simulink model "ComControleRobustoSemIntegral"  (R2024a)
settings: Solver=ode3  StartTime=0.0  StopTime=10  FixedStep=0.001  MaxStep=10^-3  RelTol=1e-6  AbsTol=10^-6
values from neighbouring files (symbols this model uses):
  A = [-807.7,  222.7,    0,      0,       0 ... (first row only)    [test.m]
  B = [-1073,  -1684,  824.5 ... (first row only)    [test.m]
  C = [21.93,  -18.87,  144.4,  -100.7,  13.85 ... (first row only)    [test.m]
undefined symbols (not defined in the file or in its folder): D, K, sigbuilder_block
libraries: simulink_extras x1
settings Model: Creator=Vilson Wenis Belle  LastModifiedBy=wenis
settings SolverCC: AlgebraicLoopSolver=TrustRegion
settings DebuggingCC: UnconnectedInputMsg=warning  UnconnectedOutputMsg=warning  UnconnectedLineMsg=warning
settings ModelReferenceCC: EnableRefExpFcnMdlSchedulingChecks=on
settings RTWCC: GPUComputeCapability=3.5  DLArmComputeVersion=19.05

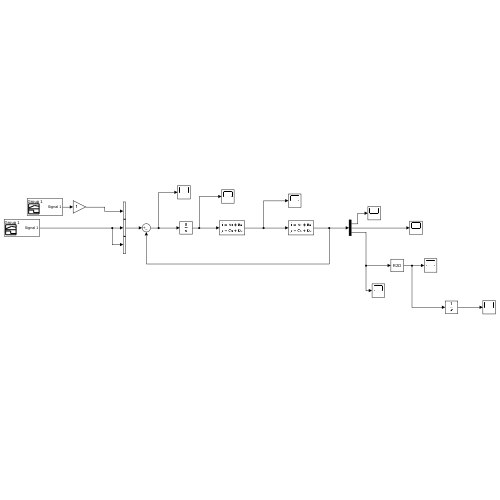
[thumbnail: Simulink's stored preview of the top-level diagram]
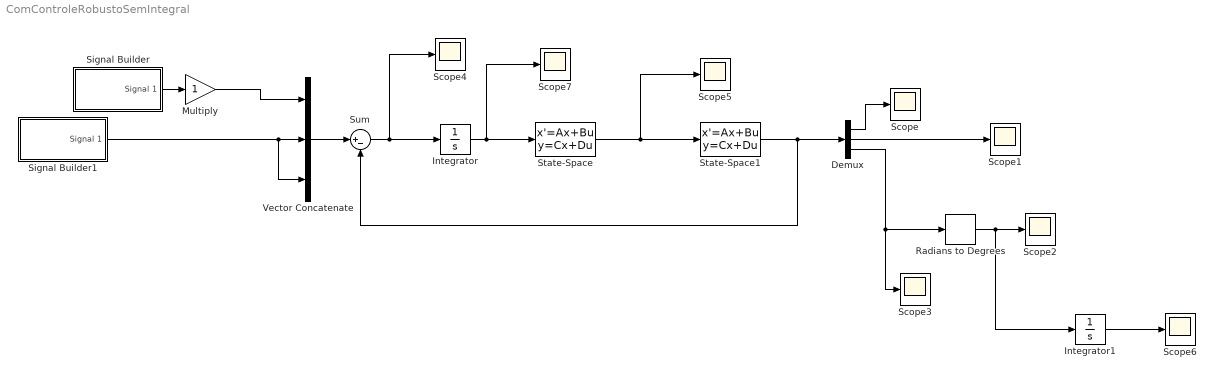
== system ComControleRobustoSemIntegral ==
  Demux : Demux  Outputs=3
  Integrator : Integrator  InitialCondition=[0 0 0]
  Integrator1 : Integrator
  Multiply : Gain
  Radians to Degrees : simulink_extras/Transformations/Radians to Degrees
  Scope{,1..7} (8 alike) : Scope
  Signal Builder : Subsystem  Tag=STV Subsys  LoadFcn=sigbuilder_block('load');  StartFcn=sigbuilder_block('start');  StopFcn=sigbuilder_block('stop');  ClipboardFcn=sigbuilder_block('clipboard');  mask(Sigbuilder block){tuvar=[0:10]}
      mask help: Simulink:masks:SigbuilderBlock_MD
      mask init:
      | if ~strcmp(get_param(bdroot(gcbh),'SimulationStatus'),'stopped') tuvar = sigbuilder_block('maskInit'); end
      settings: CopyFcn=sigbuilder_block('copy');  DeleteFcn=sigbuilder_block('delete');  ModelCloseFcn=sigbuilder_block('modelClose');  PreSaveFcn=sigbuilder_block('preSave');  PauseFcn=sigbuilder_block('pause');  ContinueFcn=sigbuilder_block('continue');  NameChangeFcn=sigbuilder_block('namechange');  OpenFcn=sigbuilder_block('open',[433.5 37.5 765.75 465.75 ]);  CloseFcn=sigbuilder_block('close');
      mask Display: plot(0, 0, 100, 100,[2, 2, 32, 32, 2], [68, 8, 8, 68, 68],[32, 2], [38, 38], [32, 19, 2],[53, 60, 44], [32, 17, 17, 2],[16, 16, 31, 31]);txt = getActiveGroup(gcbh);text(2, 100, txt,'verticalAlignment', 'top');
  Signal Builder1 : Subsystem  Tag=STV Subsys  LoadFcn=sigbuilder_block('load');  StartFcn=sigbuilder_block('start');  StopFcn=sigbuilder_block('stop');  ClipboardFcn=sigbuilder_block('clipboard');  mask(Sigbuilder block){tuvar=[0:10]}
      mask help: Simulink:masks:SigbuilderBlock_MD
      mask init:
      | if ~strcmp(get_param(bdroot(gcbh),'SimulationStatus'),'stopped') tuvar = sigbuilder_block('maskInit'); end
      settings: CopyFcn=sigbuilder_block('copy');  DeleteFcn=sigbuilder_block('delete');  ModelCloseFcn=sigbuilder_block('modelClose');  PreSaveFcn=sigbuilder_block('preSave');  PauseFcn=sigbuilder_block('pause');  ContinueFcn=sigbuilder_block('continue');  NameChangeFcn=sigbuilder_block('namechange');  OpenFcn=sigbuilder_block('open',[433.5 32.25 758.25 471 ]);  CloseFcn=sigbuilder_block('close');
      mask Display: plot(0, 0, 100, 100,[2, 2, 32, 32, 2], [68, 8, 8, 68, 68],[32, 2], [38, 38], [32, 19, 2],[53, 60, 44], [32, 17, 17, 2],[16, 16, 31, 31]);txt = getActiveGroup(gcbh);text(2, 100, txt,'verticalAlignment', 'top');
  State-Space : StateSpace  A=K.A  B=K.B  C=K.C  D=K.D  InitialCondition=[0 0 0 0 0]
  State-Space1 : StateSpace  A=A  B=B  C=C  D=D  InitialCondition=[0 0 0]
  Sum : Sum  Inputs=|+-
  Vector Concatenate : Concatenate  NumInputs=3
  wires:
  Demux/1 -> Scope/1
  Demux/2 -> Scope1/1
  State-Space1/1 -> Sum/2, Demux/1
  Demux/3 -> Scope3/1, Radians to Degrees/1
  Radians to Degrees/1 -> Integrator1/1, Scope2/1
  Sum/1 -> Integrator/1, Scope4/1
  Vector Concatenate/1 -> Sum/1
  Signal Builder1/1(Signal 1) -> Vector Concatenate/2, Vector Concatenate/3
  Integrator1/1 -> Scope6/1
  Signal Builder/1(Signal 1) -> Multiply/1
  Multiply/1 -> Vector Concatenate/1
  State-Space/1 -> Scope5/1, State-Space1/1
  Integrator/1 -> Scope7/1, State-Space/1

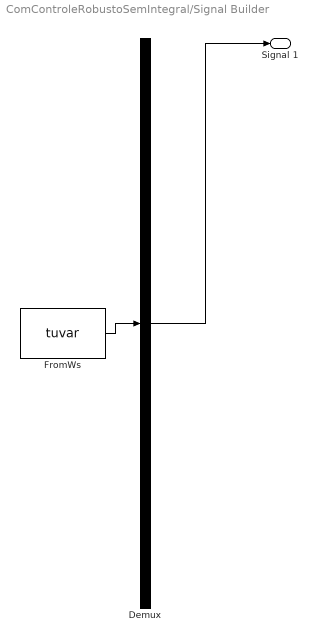
== system ComControleRobustoSemIntegral/Signal Builder ==
  Demux : Demux  Tag=STV Demux  Outputs=1
      settings: DisplayOption=none
  FromWs : FromWorkspace  Tag=STV FromWs  VariableName=tuvar
      SigBuilderData=|
      | common.afterFinalStr = 'Extrapolate'
      | common.sampleTime = 0
      | dataSet.timeRange = [0 20]
      | dataSet.name = 'Group 1'
      | sbobj.Groups.Name = 'Group 1'
      | sbobj.Groups.Signals.Name = 'Signal 1'
      | sbobj.Groups.Signals.XData = [0 1.7 1.7 20]
      | sbobj.Groups.Signals.YData = [0 0 0.5 0.5]
      | sbobj.Groups.TimeRange = [0 20]
  Signal 1 : Outport  Tag=STV Outport
  wires:
  Demux/1 -> Signal 1/1
  FromWs/1 -> Demux/1

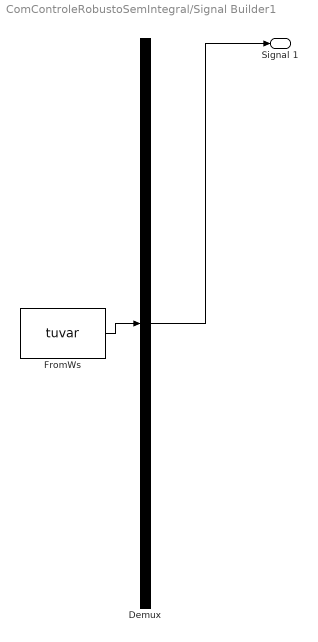
== system ComControleRobustoSemIntegral/Signal Builder1 ==
  Demux : Demux  Tag=STV Demux  Outputs=1
      settings: DisplayOption=none
  FromWs : FromWorkspace  Tag=STV FromWs  VariableName=tuvar
      SigBuilderData=|
      | common.afterFinalStr = 'Extrapolate'
      | common.sampleTime = 0
      | dataSet.timeRange = [0 20]
      | dataSet.name = 'Group 1'
      | sbobj.Groups.Name = 'Group 1'
      | sbobj.Groups.Signals.Name = 'Signal 1'
      | sbobj.Groups.Signals.XData = [0 1.7 20]
      | sbobj.Groups.Signals.YData = [0 0 0]
      | sbobj.Groups.TimeRange = [0 20]
  Signal 1 : Outport  Tag=STV Outport
  wires:
  Demux/1 -> Signal 1/1
  FromWs/1 -> Demux/1
